simulink model "Const2"  (Simulink 7.9)
settings: Solver=FixedStepDiscrete  StartTime=0.0  StopTime=100000000.0  FixedStep=1  RelTol=1e-3
settings Model: Creator=boakes  LastModifiedBy=boakes
settings OptimizationCC: BlockReduction=off  ConditionallyExecuteInputs=off  EnhancedBackFolding=on  ExpressionFolding=off

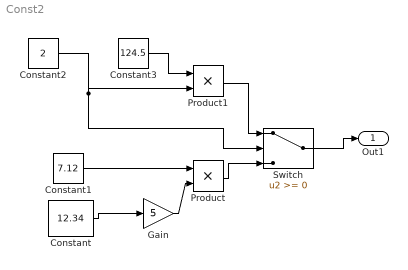
== system Const2 ==
  Constant : Constant  Value=12.34
  Constant1 : Constant  Value=7.12
  Constant2 : Constant  Value=2
  Constant3 : Constant  Value=124.5
  Gain : Gain  Gain=5
  Product : Product  RndMeth=Zero
  Product1 : Product  RndMeth=Zero
  Switch : Switch
  Out1 : Outport
  wires:
  Constant1/1 -> Product/1
  Constant/1 -> Gain/1
  Gain/1 -> Product/2
  Switch/1 -> Out1/1
  Product/1 -> Switch/3
  Constant2/1 -> Switch/2, Product1/2
  Constant3/1 -> Product1/1
  Product1/1 -> Switch/1
